simulink model "peacockElettricaSimulink"  (R2026a)
settings: Solver=FixedStepAuto  StopTime=40  FixedStep=0.001  EnableMultiTasking=on
InitFcn:
  | run('setupParams.m');
  | %run("tracks\track2.m");
StopFcn:
  | plot(out.X, out.Y);
  | axis equal;
  | grid on;
model workspace: external: MATLAB File (data not in the file)
values from neighbouring files (symbols this model uses):
  aero_bal_r = 0.5    [setupParams.m]    (also in setupParamsSingle.m)
  Af = 1.1    [setupParams.m]    (also in setupParamsSingle.m)
  auto_speed = 0    [setupParams.m]
  ay_limit = 15.0    (= 15)    [setupParams.m]    (also in setupParamsSingle.m)
  brake_bias_f = 0.40    (= 0.4)    [setupParams.m]    (also in setupParamsSingle.m = 0.6)
  brake_bias_r = 1 - brake_bias_f    (= 0.6)    [setupParams.m]    (also in setupParamsSingle.m = 0.4)
  camber_front = -1.5    [setupParams.m]    (also in setupParamsSingle.m)
  camber_rear = -1    [setupParams.m]    (also in setupParamsSingle.m)
  Cl = 1.0    (= 1)    [setupParams.m]    (also in setupParamsSingle.m)
  deathzone_APP = 5    [setupParams.m]    (also in setupParamsSingle.m)
  e_yaw_deadzone = 0.03    [setupParams.m]
  falling_slew_rate_torque = -500    [setupParams.m]    (also in setupParamsSingle.m)
  g = 9.81    [setupParams.m]    (also in setupParamsSingle.m)
  gnd_displ = 0.0    (= 0)    [setupParams.m]    (also in setupParamsSingle.m)
  h_o = 0.35    [setupParams.m]    (also in setupParamsSingle.m)
  I_charge_max = 21    [setupParams.m]
  I_discharge_max = 90    [setupParams.m]
  K_roll_rear = 0.6    [setupParams.m]    (also in setupParamsSingle.m = 0.5)
  Kus = 0.03    [setupParams.m]    (also in setupParamsSingle.m = 0)
  l_f = 0.775    [setupParams.m]    (also in setupParamsSingle.m)
  l_r = 0.775    [setupParams.m]    (also in setupParamsSingle.m)
  launch_ramp_rate = 1000.0    (= 1000)    [setupParams.m]    (also in setupParamsSingle.m)
  launch_V_thresh = 5.0    (= 5)    [setupParams.m]    (also in setupParamsSingle.m)
  mass = 320    [setupParams.m]    (also in setupParamsSingle.m = 300)
  mu = 1.5    [setupParams.m]    (also in setupParamsSingle.m)
  nominal_ramp_rate = 1000.0    (= 1000)    [setupParams.m]    (also in setupParamsSingle.m)
  overslip_factor = 1.01    [setupParams.m]    (also in setupParamsSingle.m = 1.13)
  pa_front_wheel = 82700    [setupParams.m]    (also in setupParamsSingle.m)
  pa_rear_wheel = 82700    [setupParams.m]    (also in setupParamsSingle.m)
  pedal_bp = (0:10:100)'    [setupParams.m]    (also in setupParamsSingle.m)
  pedal_map = (pedal_bp / 100) .^ pedal_alpha    [setupParams.m]    (also in setupParamsSingle.m = (pedal_bp / 100) .^ pedal_alpha.Value)
  R_wheel = 0.2032    [setupParams.m]    (also in setupParamsSingle.m)
  regen_I_cont_A = 14.0    (= 14)    [setupParams.m]    (also in setupParamsSingle.m)
  regen_I_peak_A = 21.0    (= 21)    [setupParams.m]    (also in setupParamsSingle.m)
  regen_I_peak_dur_s = 4.0    (= 4)    [setupParams.m]    (also in setupParamsSingle.m)
  regen_P_batt_max_W = 35000    [setupParams.m]    (also in setupParamsSingle.m)
  regen_pedal_thr = 5.0    (= 5)    [setupParams.m]    (also in setupParamsSingle.m = 10)
  regen_speed_crit_rpm = 1000    [setupParams.m]    (also in setupParamsSingle.m = 500)
  regen_speed_min_rpm = 4000    [setupParams.m]    (also in setupParamsSingle.m = 3000)
  regen_T_max = 9    [setupParams.m]    (also in setupParamsSingle.m = Simulink.Parameter(T_rated.Value/2))
  rho = 1.225    [setupParams.m]    (also in setupParamsSingle.m)
  rid_eff = 0.80    (= 0.8)    [setupParams.m]    (also in setupParamsSingle.m)
  rid_ratio = 15    [setupParams.m]    (also in setupParamsSingle.m)
  rising_slew_rate_torque = 100    [setupParams.m]    (also in setupParamsSingle.m)
  rpm_safe_threshold = 100    [setupParams.m]
  scale_factor_front = ones(27, 1)    [setupParams.m]    (also in setupParamsSingle.m)
  scale_factor_rear = ones(27, 1)    [setupParams.m]    (also in setupParamsSingle.m)
  slip_bc_coeff = 10    [setupParams.m]    (also in setupParamsSingle.m = Simulink.Parameter(1.5))
  slip_filt_N = 80    [setupParams.m]    (also in setupParamsSingle.m = 15)
  slip_Kd = 0.8    [setupParams.m]    (also in setupParamsSingle.m = Simulink.Parameter(5.0))
  slip_Ki = 13.0    (= 13)    [setupParams.m]    (also in setupParamsSingle.m = Simulink.Parameter(110.0))
  slip_Kp = 50.0    (= 50)    [setupParams.m]    (also in setupParamsSingle.m = Simulink.Parameter(180.0))
  slip_low_sat = 0.0    (= 0)    [setupParams.m]    (also in setupParamsSingle.m)
  slip_ref = 0.15    [setupParams.m]    (also in setupParamsSingle.m = Simulink.Parameter(0.15))
  slip_up_sat = 25    [setupParams.m]    (also in setupParamsSingle.m = 21)
  slip_V_min = 3    [setupParams.m]    (also in setupParamsSingle.m = 1)
  steer_ratio = 4.2    [pure_pursuit.m]    (also in setupParams.m; setupParamsSingle.m)
  steering_deadband = 1    [setupParams.m]
  T_headroom_k = 13.0    (= 13)    [setupParams.m]    (also in setupParamsSingle.m = Simulink.Parameter(5.0))
  T_headroom_max = 9    [setupParams.m]    (also in setupParamsSingle.m = Simulink.Parameter(5.0))
  T_peak = 20    [setupParams.m]    (also in setupParamsSingle.m = 21)
  T_rated = 9.8    [setupParams.m]    (also in setupParamsSingle.m = Simulink.Parameter(9.8))
  track_width = (track_width_r + track_width_f)/2    (= 1.2)    [setupParams.m]    (also in setupParamsSingle.m = sqrt(track_width_r^2 + track_width_f^2))
  track_width_f = 1.2    [setupParams.m]    (also in setupParamsSingle.m)
  track_width_r = 1.2    [setupParams.m]    (also in setupParamsSingle.m)
  Ts = 0.01    [setupParams.m]    (also in setupParamsSingle.m)
  tvc_bc = 17    [setupParams.m]
  tvc_D_thresh = 0.060    (= 0.06)    [setupParams.m]    (also in setupParamsSingle.m)
  tvc_D_thresh_off = 0.03    [setupParams.m]    (also in setupParamsSingle.m)
  tvc_Kd = 100    [setupParams.m]    (also in setupParamsSingle.m = Simulink.Parameter(5))
  tvc_Ki = 150    [setupParams.m]    (also in setupParamsSingle.m = Simulink.Parameter(10))
  tvc_Kp = 650    [setupParams.m]    (also in setupParamsSingle.m = Simulink.Parameter(70))
  tvc_N_filter = 25    [setupParams.m]    (also in setupParamsSingle.m = Simulink.Parameter(20))
  tvc_sat_dMz = 700    [setupParams.m]    (also in setupParamsSingle.m = Simulink.Parameter(10.0))
  tvc_throttle_on = 3.0    (= 3)    [setupParams.m]    (also in setupParamsSingle.m = Simulink.Parameter(3.0))
  tvc_tr = 5    [setupParams.m]    (also in setupParamsSingle.m = Simulink.Parameter(1.0))
  tvc_V_off = 2.0    (= 2)    [setupParams.m]    (also in setupParamsSingle.m = Simulink.Parameter(2.0))
  tvc_V_on = 4.0    (= 4)    [setupParams.m]    (also in setupParamsSingle.m = Simulink.Parameter(4.0))
  tvc_yaw_thresh = 0.08    [setupParams.m]    (also in setupParamsSingle.m)
  tvc_yaw_thresh_off = 0.04    [setupParams.m]    (also in setupParamsSingle.m)
  V_dc = 540    [setupParams.m]    (also in setupParamsSingle.m)
  w_engine = 0.005    [setupParams.m]    (also in setupParamsSingle.m)
  wheelbase = l_f + l_r    (= 1.55)    [setupParams.m]    (also in setupParamsSingle.m)
undefined symbols (not defined in the file or in its folder): V_ref, X_ref, Y_ref
libraries: simulink x74, slpidlib x8, vehdynlibtire x8, dspsigops x4, vehdynlibsteering x2, autolibshared x2, sim3dautolib x2, sim3dlib x1, robotalgslib x1
(part 6 of 6)

== matlab function peacockElettricaSimulink/DriveController_/TVC/TorqueAllocator ==
  data: T_req input; T_RL_cmd output; dT input; n_motorRL input; n_motorRR input; T_RR_cmd output; D input; V_dc parameter; T_peak parameter; T_headroom_max parameter; T_headroom_k parameter; T_grip_max_RL input; T_grip_max_RR input; rpm_safe_threshold parameter; I_discharge_max parameter
function [T_RL_cmd, T_RR_cmd] = fcn(T_req, dT, n_motorRL, n_motorRR, D, ...
    V_dc, T_peak, T_headroom_max, T_headroom_k, T_grip_max_RL, T_grip_max_RR, rpm_safe_threshold, I_discharge_max)
    T_min = 0;
    
    % --- CALCOLO POTENZA MASSIMA (Inverter) ---
    P_max_inverter = V_dc * 58.33; 
    
    % --- CALCOLO LIMITI ELETTRICI (FIELD WEAKENING) ---
    w_RL = max(abs(n_motorRL) * (pi/30), 1.0); 
    w_RR = max(abs(n_motorRR) * (pi/30), 1.0);
    
    T_fw_L = P_max_inverter / w_RL;
    T_fw_R = P_max_inverter / w_RR;
    
    T_elec_max_RL = min(T_peak, T_fw_L);
    T_elec_max_RR = min(T_peak, T_fw_R);
    
    % --- LIMITI FISICI GLOBALI ---
    T_max_L = min(T_elec_max_RL, T_grip_max_RL);
    T_max_R = min(T_elec_max_RR, T_grip_max_RR);
    
    % ---  PROTEZIONE ASIMMETRIA E HEADROOM TVC ---
    T_lim_base = min(T_max_L, T_max_R);
    T_headroom = min(T_headroom_max, T_headroom_k * abs(D));
    
    T_lim_base_neg = -min(T_grip_max_RL, T_grip_max_RR); 
    
    if T_req >= 0
        T_req_eff = max(0, min(T_req, T_lim_base - T_headroom));
    else
        T_req_eff = max(T_lim_base_neg + T_headroom, min(0, T_req));
    end
    
    % ---  TEORICO TVC ---
    T_L = T_req_eff - dT;
    T_R = T_req_eff + dT;
    
    if (abs(n_motorRL) < rpm_safe_threshold) && (T_L < 0)
        T_L = 0;
    end
    if (abs(n_motorRR) < rpm_safe_threshold) && (T_R < 0)
        T_R = 0;
    end
    
    % --- LIMITAZIONE PROPORZIONALE POTENZA DC (DC Current Limit) ---
    P_req_L = max(0, T_L * w_RL);
    P_req_R = max(0, T_R * w_RR);
    P_tot_req = P_req_L + P_req_R;
    
    P_limit_dc = V_dc * I_discharge_max;
    
    if P_tot_req > P_limit_dc
        scale_factor = P_limit_dc / P_tot_req;
        T_L = T_L * scale_factor;
        T_R = T_R * scale_factor;
    end
    
    % --- SATURAZIONE FINALE ---
    T_RL_cmd = max(-T_grip_max_RL, min(T_max_L, T_L));
    T_RR_cmd = max(-T_grip_max_RR, min(T_max_R, T_R));
end

== matlab function peacockElettricaSimulink/G_motor_RR/MATLAB Function ==
  data: T_thermal input; T_req input; derating_out output; derating_prev input; derating_on_thresh parameter
% function derating_out = fcn(T_thermal, derating_prev,T_peak, derating_on_thresh, derating_off_thresh)
%     if derating_prev == 0
%         % Se il limite termico cala troppo, attivo il flag
%         derating_out = double(T_thermal < derating_on_thresh);
%     else
%         % Resto in derating finché il limite non ha recuperato abbastanza
%         derating_out = double(T_thermal < derating_off_thresh);
%     end
% end

function derating_out = fcn(T_thermal, T_req, derating_prev,derating_on_thresh)

if derating_prev == 0
    % Se NON sono in derating, controllo se devo entrarci
    if T_thermal < derating_on_thresh
        derating_out = 1;
    else
        derating_out = 0;
    end
else
    if T_req <= 1 % Uso un piccolo margine invece di 0 spaccato per robustezza numerica
        derating_out = 0; % Esco dal derating
    else
        derating_out = 1; % Mantengo il derating
    end
end
end

== matlab function peacockElettricaSimulink/DriveController_/Yaw_th/tand safe ==
  data: tand input; tand_safe output; angle_limit_d parameter
function tand_safe = fcn(tand,angle_limit_d)
    soglia = tan(angle_limit_d*pi/180);  % 2° rad
    
    if abs(tand) < soglia
        tand_safe = 0;  % 
    else
        tand_safe = tand;  
    end
end

== matlab function peacockElettricaSimulink/DriveController_/Yaw_th/yaw_saturation ==
  data: yaw_th input; yaw_sat output; V input; mu parameter; g parameter
function yaw_sat = fcn(yaw_th, V,mu, g)
    V_calc = max(V, 0.5);
    
    yaw_max_abs = (mu * g) / V_calc;
    yaw_sat = sign(yaw_th) * min(abs(yaw_th), yaw_max_abs);
end

== matlab function peacockElettricaSimulink/DriveController_/SRC/MATLAB Function ==
  data: enable input; T_cut_RL output; Delta_T_raw input
function T_cut_RL = fcn(enable, Delta_T_raw)
    T_cut_RL = enable * Delta_T_raw;
end

== matlab function peacockElettricaSimulink/DriveController_/SRC/MATLAB Function1 ==
  data: enable input; T_cut_RR output; Delta_T_raw input
function T_cut_RR = fcn(enable, Delta_T_raw)
    T_cut_RR = enable * Delta_T_raw;
end

== matlab function peacockElettricaSimulink/PeacockElettrica_/MATLAB Function1 ==
  data: Vx input; Vx_hub output; Vy input; yaw input; delta_L input; delta_R input; Vy_hub output; track_width_f parameter; track_width_r parameter; l_f parameter; l_r parameter
function [Vx_hub, Vy_hub] = wheel_kinematics(Vx, Vy, yaw, delta_L, delta_R, track_width_f, track_width_r, l_f, l_r)
% Trasforma le velocità del baricentro (CG) nelle velocità locali dei mozzi ruota.
%
% INPUTS:
% Vx, Vy  : Velocità longitudinali e laterali del veicolo (CG) [m/s]
% yaw       : Velocità di imbardata (Yaw rate) [rad/s]
% delta_L : Angolo di sterzo ruota anteriore sinistra [rad]
% delta_R : Angolo di sterzo ruota anteriore destra [rad]
% l_f, l_r: Distanza baricentro - asse anteriore/posteriore [m]
% track_width_f, track_width_r: Carreggiata (Track width) anteriore/posteriore [m]
%
% OUTPUTS:
% Vx_hub  : Vettore [FL, FR, RL, RR] delle velocità longitudinali dei mozzi [m/s]
% Vy_hub  : Vettore [FL, FR, RL, RR] delle velocità laterali dei mozzi [m/s]

    %% 1. Velocità nel sistema di riferimento del telaio (non ruotate)
    % Anteriore Sinistra (Front Left)
    V_xf_FL = Vx - (yaw * track_width_f / 2);
    V_yf_FL = Vy + (yaw * l_f);
    
    % Anteriore Destra (Front Right)
    V_xf_FR = Vx + (yaw * track_width_f / 2);
    V_yf_FR = Vy + (yaw * l_f);
    
    % Posteriore Sinistra (Rear Left)
    V_xr_RL = Vx - (yaw * track_width_r / 2);
    V_yr_RL = Vy - (yaw * l_r);
    
    % Posteriore Destra (Rear Right)
    V_xr_RR = Vx + (yaw * track_width_r / 2);
    V_yr_RR = Vy - (yaw * l_r);

    %% 2. Rotazione nel sistema di riferimento della gomma (tramite angolo di sterzo)
    % Le ruote anteriori sono sterzanti
    Vx_FL =  V_xf_FL * cos(delta_L) + V_yf_FL * sin(delta_L);
    Vy_FL = -V_xf_FL * sin(delta_L) + V_yf_FL * cos(delta_L);
    
    Vx_FR =  V_xf_FR * cos(delta_R) + V_yf_FR * sin(delta_R);
    Vy_FR = -V_xf_FR * sin(delta_R) + V_yf_FR * cos(delta_R);
    
    % Le ruote posteriori solitamente non sterzano (delta = 0, quindi cos(0)=1, sin(0)=0)
    Vx_RL = V_xr_RL;
    Vy_RL = V_yr_RL;
    
    Vx_RR = V_xr_RR;
    Vy_RR = V_yr_RR;

    Vx_hub = [Vx_FL; Vx_FR; Vx_RL; Vx_RR];
    Vy_hub = [Vy_FL; Vy_FR; Vy_RL; Vy_RR];
end

== matlab function peacockElettricaSimulink/DriveController_/MATLAB Function ==
  settings: updateMethod=DISCRETE
  data: throttle_pct input; T_regen output; n_motorRL input; n_motorRR input; V input; regen_active output; Ts parameter; regen_T_max parameter; regen_pedal_thr parameter; regen_speed_min_rpm parameter; regen_speed_crit_rpm parameter; regen_I_peak_A parameter; regen_I_cont_A parameter; regen_I_peak_dur_s parameter; regen_P_batt_max_W parameter; V_dc parameter; ay input; ay_limit parameter; I_charge_max parameter
function [T_regen, regen_active] = regen_fcn( ...
        throttle_pct, n_motorRL, n_motorRR, V, Ts, ...
        regen_T_max, regen_pedal_thr, regen_speed_min_rpm, regen_speed_crit_rpm, ...
        regen_I_peak_A, regen_I_cont_A, regen_I_peak_dur_s, ...
        regen_P_batt_max_W, V_dc, ay, ay_limit, I_charge_max)

    persistent t_elapsed_s;
    if isempty(t_elapsed_s)
        t_elapsed_s = 0.0;
    end
    speed_avg_rpm = (abs(n_motorRL) + abs(n_motorRR)) * 0.5;
    
    % ---- condizione di abilitazione regen 
    should_regen = (throttle_pct <= regen_pedal_thr) && ...
                   (speed_avg_rpm > regen_speed_crit_rpm) && ...
                   (V > 0.5);
    if ~should_regen
        t_elapsed_s = 0.0;
        T_regen = 0;
        regen_active = 0.0;
        return;
    end
    
    t_elapsed_s = t_elapsed_s + Ts;
    
    % ---- Stage 1: coppia pedal-dipendente [Nm, negativa] ----------------
    pedal_norm = throttle_pct / regen_pedal_thr;
    T_s1 = -regen_T_max * (1.0 - pedal_norm);
    
    % ---- Stage 2: fade-out velocità -------------------------------------
    if speed_avg_rpm >= regen_speed_min_rpm
        k_vel = 1.0;
    else
        k_vel = speed_avg_rpm / regen_speed_min_rpm;
    end
    T_s2 = T_s1 * k_vel;
    
    % ---- Stage 3: limite potenza batteria (per motore = totale/2) -------
    omega_rad_s = (2.0 * pi * speed_avg_rpm) / 60.0;
    omega_safe  = max(omega_rad_s, 1.0);          
    T_P_lim     = (regen_P_batt_max_W * 0.5) / omega_safe;
    T_s3        = max(T_s2, -T_P_lim);            
    
    % --- NUOVO: INCROCIO LIMITI DI CORRENTE BMS ---
    if t_elapsed_s < regen_I_peak_dur_s
        I_lim_teorico = regen_I_peak_A;    
    else
        I_lim_teorico = regen_I_cont_A;   
    end
    
    % Sceglie il limite più severo tra la logica timer e il CAN del BMS
    I_lim_effettivo = min(I_lim_teorico, I_charge_max);
    I_lim_per_mot = I_lim_effettivo * 0.5;
    
    T_I_lim = (I_lim_per_mot * V_dc) / omega_safe;
    T_final = max(T_s3, -T_I_lim);
    
    % ---- Stage 4: limite regen x curva ----------------------------------
    k_derating_ay = max(0.0, 1.0 - (abs(ay) / ay_limit));
    T_final = T_final * k_derating_ay;
    
    % ---- output simmetrico sui due motori -------------------------------
    T_regen  = T_final;
    regen_active = 1; 
end

== matlab function peacockElettricaSimulink/DriveController_/MATLAB Function1 ==
  data: T_max_RL output; v_x input; a_x input; a_y input; T_max_RR output; mass parameter; g parameter; wheelbase parameter; l_f parameter; track_width_r parameter; mu parameter; h_o parameter; R_wheel parameter; Af parameter; Cl parameter; aero_bal_r parameter; K_roll_rear parameter; rho parameter; rid_ratio parameter; rid_eff parameter; overslip_factor parameter
function [T_max_RL, T_max_RR] = GripEstimator(v_x, a_x, a_y, mass, g, wheelbase, l_f, track_width_r,mu,h_o, R_wheel,Af, Cl, aero_bal_r, K_roll_rear, rho, rid_ratio,rid_eff, overslip_factor)
    % ---------------------------------------------------------
    % 1. CARICO BASE (Statico + Aerodinamico)
    % ---------------------------------------------------------
    Fz_stat_rear = mass * g * (l_f / wheelbase);
    
    Fz_aero_rear = 0.5 * rho * Af * Cl * (v_x^2) * aero_bal_r;
    
    Fz_base_wheel = (Fz_stat_rear + Fz_aero_rear) / 2;

   
    % 2. TRASFERIMENTI DI CARICO
    % Longitudinale: se a_x > 0 (accelerazione), il peso si sposta dietro (+)
    delta_Fz_long = 0.5 * (mass * a_x * h_o / wheelbase);
    
    % Laterale: dipende dall'accelerazione laterale a_y.
    % Convenzione: a_y < 0 per curva a destra-> peso si sposta a sinistra.
    delta_Fz_lat = (mass * a_y * h_o / track_width_r) * K_roll_rear;

    % 3. FORZE NORMALI FINALI SULLE RUOTE (Fz)
    Fz_RL = Fz_base_wheel + delta_Fz_long + delta_Fz_lat;
    Fz_RR = Fz_base_wheel + delta_Fz_long - delta_Fz_lat;

    % Prevenzione valori negativi (se la ruota interna si alza da terra, Fz = 0)
    if Fz_RL < 0
        Fz_RL = 0;
    end
    if Fz_RR < 0
        Fz_RR = 0;
    end
    

    
    % 4. CALCOLO COPPIA MASSIMA AI MOTORI
    % T = (F * R) / (tau * eff)

    % Parametri Pacejka (dal file .tir)
    Fz0 = 1112.0;
    PDX1 = 1.00347;
    PDX2 = -0.99198;

    % Calcolo mu dinamico per lato sinistro
    dfz_RL = (Fz_RL - Fz0) / Fz0;
    mu_RL = PDX1 + (PDX2 * dfz_RL);
    
    % Saturazione di sicurezza (evita mu negativi o assurdi)
    if mu_RL < 0.5; mu_RL = 0.5; end

    % Calcolo mu dinamico per lato destro
    dfz_RR = (Fz_RR - Fz0) / Fz0;
    mu_RR = PDX1 + (PDX2 * dfz_RR);
    if mu_RR < 0.5; mu_RR = 0.5; end
    
   

    % % Calcolo coppia massima ai motori usando il mu corretto
    % T_max_RL = (Fz_RL * mu_RL * R_wheel) / (rid_ratio * rid_eff);
    % T_max_RR = (Fz_RR * mu_RR * R_wheel) / (rid_ratio * rid_eff);

    % Calcolo coppia massima ai motori
     %T_max_RL = ((Fz_RL * mu_RL * R_wheel) / (rid_ratio * rid_eff)) * overslip_factor;
     %T_max_RR = ((Fz_RR * mu_RR * R_wheel) / (rid_ratio * rid_eff)) * overslip_factor;

    T_max_RL = (Fz_RL * mu * R_wheel) / (rid_ratio * rid_eff)* overslip_factor;
    T_max_RR = (Fz_RR * mu * R_wheel) / (rid_ratio * rid_eff)* overslip_factor;
end

== matlab function peacockElettricaSimulink/G_motor_RR/MATLAB Function1 ==
  data: rpm_motor input; T_limit output; V_dc input
function T_limit = fcn(rpm_motor, V_dc)
    %potenza massima erogabile: 35kW(max) / 600V = 58.33
    P_max = V_dc * 58.33; 

    w_rad = max(abs(rpm_motor) * (pi/30), 1.0); 

    T_limit = P_max / w_rad;
end

== matlab function peacockElettricaSimulink/G_motor_RL/Field weakening ==
  data: rpm_motor input; T_limit output; V_dc input
function T_limit = fcn(rpm_motor, V_dc)
    P_max = V_dc * 58.33; 

    w_rad = max(abs(rpm_motor) * (pi/30), 1.0); 

    T_limit = P_max / w_rad;
end

== matlab function peacockElettricaSimulink/PeacockElettrica_/MATLAB Function ==
  data: Fx_FL input; FwF output; Fy_FL input; Fx_FR input; Fy_FR input; Fx_RL input; Fy_RL input; Fx_RR input; Fy_RR input; delta_L input; FwR output; delta_R input
function [FwF, FwR] = rotazione_forze(Fx_FL, Fy_FL, Fx_FR, Fy_FR, Fx_RL, Fy_RL, Fx_RR, Fy_RR, delta_L, delta_R)
    
    % 1. Ruota le forze della ruota Anteriore Sinistra (FL) usando l'angolo sinistro (delta_L)
    Fx_veh_FL = Fx_FL * cos(delta_L) - Fy_FL * sin(delta_L);
    Fy_veh_FL = Fx_FL * sin(delta_L) + Fy_FL * cos(delta_L);

    % 2. Ruota le forze della ruota Anteriore Destra (FR) usando l'angolo destro (delta_R)
    Fx_veh_FR = Fx_FR * cos(delta_R) - Fy_FR * sin(delta_R);
    Fy_veh_FR = Fx_FR * sin(delta_R) + Fy_FR * cos(delta_R);

    % 3. Crea la matrice 2x2 per la porta FwF (Asse Anteriore)
    FwF = [Fx_veh_FL, Fy_veh_FL;
           Fx_veh_FR, Fy_veh_FR];

    % 4. Crea la matrice 2x2 per la porta FwR (Asse Posteriore)
    % (Le posteriori non sterzano, quindi i valori rimangono quelli originali della gomma)
    FwR = [Fx_RL, Fy_RL;
           Fx_RR, Fy_RR];
end

== matlab function peacockElettricaSimulink/MATLAB Function ==
  data: curv input; v_curv output; a_lat_max parameter
function v_curv = fcn(curv,a_lat_max)

v_curv_raw = sqrt(a_lat_max / (abs(curv)+0.001));

v_curv = min(v_curv_raw, 100);

== matlab function peacockElettricaSimulink/Target Velocity Profiler ==
  data: x input; V_target output; y input; lookahead_pts input; X_ref parameter; Y_ref parameter; V_ref parameter
function V_target = fcn(x, y, lookahead_pts, X_ref, Y_ref, V_ref)
    % V_TARGET_PROFILER Trova la velocità target in base alla posizione
    % X_ref, Y_ref, V_ref_array devono essere passati come Parametri (o segnali) di dimensione [1x1500]
    
    % 1. Calcola la distanza quadrata tra l'auto e tutti i punti della traiettoria
    dist_sq = (X_ref - x).^2 + (Y_ref - y).^2;
    
    % 2. Trova l'indice del punto più vicino sulla pista
    [~, current_idx] = min(dist_sq);
    
    % 3. Look-ahead della velocità (FONDAMENTALE PER LA FRENATA)
    % Se chiedi all'auto di rallentare quando è GIA' nel punto di corda, andrà dritta.
    % Dobbiamo dirle di guardare la velocità dei punti successivi per iniziare a frenare prima.
    target_idx = current_idx + lookahead_pts;
    
    % Gestione della chiusura del tracciato (loop)
    num_points = length(X_ref);
    if target_idx > num_points
        target_idx = target_idx - num_points; 
    end
    
    % 4. Estrai la velocità di riferimento
    V_target = V_ref(target_idx);
end

== matlab function peacockElettricaSimulink/PeacockElettrica/Car Body/MATLAB Function ==
  data: delta_L input; delta_R input; Fx_FL input; FwF output; Fy_FL input; Fx_FR input; Fy_FR input; Fx_RL input; Fy_RL input; Fx_RR input; Fy_RR input; FwR output
function [FwF, FwR] = rotationary_forces(delta_L, delta_R, Fx_FL, Fy_FL, Fx_FR, Fy_FR, Fx_RL, Fy_RL, Fx_RR, Fy_RR)
    
    % 1. Ruota le forze della ruota Anteriore Sinistra (FL) usando l'angolo sinistro (delta_L)
    Fx_veh_FL = Fx_FL * cos(delta_L) - Fy_FL * sin(delta_L);
    Fy_veh_FL = Fx_FL * sin(delta_L) + Fy_FL * cos(delta_L);

    % 2. Ruota le forze della ruota Anteriore Destra (FR) usando l'angolo destro (delta_R)
    Fx_veh_FR = Fx_FR * cos(delta_R) - Fy_FR * sin(delta_R);
    Fy_veh_FR = Fx_FR * sin(delta_R) + Fy_FR * cos(delta_R);


FwF = [Fx_veh_FL, -Fy_veh_FL;
       Fx_veh_FR, -Fy_veh_FR];

FwR = [Fx_RL, -Fy_RL;
       Fx_RR, -Fy_RR];
end

== matlab function peacockElettricaSimulink/DriveController_/TVC/MATLAB Function ==
  data: dMz input; dT output; R_wheel parameter; track_width parameter; rid_ratio parameter; rid_eff parameter
function dT = fcn(dMz, R_wheel, track_width, rid_ratio, rid_eff)
    dT = dMz * R_wheel / (track_width * rid_ratio * rid_eff);
end

== matlab function peacockElettricaSimulink/PeacockElettrica/Car Body/car2wheels ==
  data: delta_L input; delta_R input; Vx input; Vx_hub output; Vy input; yaw_rate input; Vy_hub output; track_width_f parameter; track_width_r parameter; l_f parameter; l_r parameter
function [Vx_hub, Vy_hub] = wheel_kinematics(delta_L, delta_R, Vx, Vy, yaw_rate, track_width_f, track_width_r, l_f, l_r)
% Trasforma le velocità del baricentro (CG) nelle velocità locali dei mozzi ruota.
%
% INPUTS:
% Vx, Vy  : Velocità longitudinali e laterali del veicolo (CG) [m/s]
% yaw_rate       : Velocità di imbardata (yaw_rate ) [rad/s]
% delta_L : Angolo di sterzo ruota anteriore sinistra [rad]
% delta_R : Angolo di sterzo ruota anteriore destra [rad]
% l_f, l_r: Distanza baricentro - asse anteriore/posteriore [m]
% track_width_f, track_width_r: Carreggiata (Track width) anteriore/posteriore [m]
%
% OUTPUTS:
% Vx_hub  : Vettore [FL, FR, RL, RR] delle velocità longitudinali dei mozzi [m/s]
% Vy_hub  : Vettore [FL, FR, RL, RR] delle velocità laterali dei mozzi [m/s]

    %% 1. Velocità nel sistema di riferimento del telaio (non ruotate)
    % Anteriore Sinistra (Front Left)
    V_xf_FL = Vx - (yaw_rate * track_width_f / 2);
    V_yf_FL = Vy + (yaw_rate * l_f);
    
    % Anteriore Destra (Front Right)
    V_xf_FR = Vx + (yaw_rate * track_width_f / 2);
    V_yf_FR = Vy + (yaw_rate * l_f);
    
    % Posteriore Sinistra (Rear Left)
    V_xr_RL = Vx - (yaw_rate * track_width_r / 2);
    V_yr_RL = Vy - (yaw_rate * l_r);
    
    % Posteriore Destra (Rear Right)
    V_xr_RR = Vx + (yaw_rate * track_width_r / 2);
    V_yr_RR = Vy - (yaw_rate * l_r);

    %% 2. Rotazione nel sistema di riferimento della gomma (tramite angolo di sterzo)
    % Le ruote anteriori sono sterzanti
    Vx_FL =  V_xf_FL * cos(delta_L) + V_yf_FL * sin(delta_L);
    Vy_FL = -V_xf_FL * sin(delta_L) + V_yf_FL * cos(delta_L);
    
    Vx_FR =  V_xf_FR * cos(delta_R) + V_yf_FR * sin(delta_R);
    Vy_FR = -V_xf_FR * sin(delta_R) + V_yf_FR * cos(delta_R);
    
    % Le ruote posteriori solitamente non sterzano (delta = 0, quindi cos(0)=1, sin(0)=0)
    Vx_RL = V_xr_RL;
    Vy_RL = V_yr_RL;
    
    Vx_RR = V_xr_RR;
    Vy_RR = V_yr_RR;

    Vx_hub = [Vx_FL; Vx_FR; Vx_RL; Vx_RR];
    Vy_hub = [Vy_FL; Vy_FR; Vy_RL; Vy_RR];
end

== matlab function peacockElettricaSimulink/PeacockElettrica/G_motor_RL/Derating ==
  data: T_thermal input; T_req input; derating_out output; derating_prev input; derating_on_thresh parameter
function derating_out = fcn(T_thermal, T_req, derating_prev,derating_on_thresh)

if derating_prev == 0
    % Se NON sono in derating, controllo se devo entrarci
    if T_thermal < derating_on_thresh
        derating_out = 1;
    else
        derating_out = 0;
    end
else
    if T_req <= 1 % Uso un piccolo margine invece di 0 spaccato per robustezza numerica
        derating_out = 0; % Esco dal derating
    else
        derating_out = 1; % Mantengo il derating
    end
end
end

== matlab function peacockElettricaSimulink/PeacockElettrica/G_motor_RL/Field weakening ==
  data: rpm_motor input; T_limit output; V_dc input
function T_limit = fcn(rpm_motor, V_dc)
    P_max = V_dc * 58.33; 

    w_rad = max(abs(rpm_motor) * (pi/30), 1.0); 

    T_limit = P_max / w_rad;
end

== matlab function peacockElettricaSimulink/PeacockElettrica/G_motor_RR/MATLAB Function ==
  data: T_thermal input; T_req input; derating_out output; derating_prev input; derating_on_thresh parameter
% function derating_out = fcn(T_thermal, derating_prev,T_peak, derating_on_thresh, derating_off_thresh)
%     if derating_prev == 0
%         % Se il limite termico cala troppo, attivo il flag
%         derating_out = double(T_thermal < derating_on_thresh);
%     else
%         % Resto in derating finché il limite non ha recuperato abbastanza
%         derating_out = double(T_thermal < derating_off_thresh);
%     end
% end

function derating_out = fcn(T_thermal, T_req, derating_prev,derating_on_thresh)

if derating_prev == 0
    % Se NON sono in derating, controllo se devo entrarci
    if T_thermal < derating_on_thresh
        derating_out = 1;
    else
        derating_out = 0;
    end
else
    if T_req <= 1 % Uso un piccolo margine invece di 0 spaccato per robustezza numerica
        derating_out = 0; % Esco dal derating
    else
        derating_out = 1; % Mantengo il derating
    end
end
end

== matlab function peacockElettricaSimulink/PeacockElettrica/G_motor_RR/MATLAB Function1 ==
  data: rpm_motor input; T_limit output; V_dc input
function T_limit = fcn(rpm_motor, V_dc)
    %potenza massima erogabile: 35kW(max) / 600V = 58.33
    P_max = V_dc * 58.33; 

    w_rad = max(abs(rpm_motor) * (pi/30), 1.0); 

    T_limit = P_max / w_rad;
end

== matlab function peacockElettricaSimulink/PeacockElettrica/Car Body/V ==
  data: Vx input; V output; Vy input
function V = fcn(Vx,Vy)

V = (Vx^2 + Vy^2)^0.5;

== matlab function peacockElettricaSimulink/DriveController/MATLAB Function ==
  settings: updateMethod=DISCRETE
  data: throttle_pct input; T_regen output; n_motorRL input; n_motorRR input; V input; regen_active output; Ts parameter; regen_T_max parameter; regen_pedal_thr parameter; regen_speed_min_rpm parameter; regen_speed_crit_rpm parameter; regen_I_peak_A parameter; regen_I_cont_A parameter; regen_I_peak_dur_s parameter; regen_P_batt_max_W parameter; V_dc parameter; ay input; ay_limit parameter; I_charge_max parameter
function [T_regen, regen_active] = regen_fcn( ...
        throttle_pct, n_motorRL, n_motorRR, V, Ts, ...
        regen_T_max, regen_pedal_thr, regen_speed_min_rpm, regen_speed_crit_rpm, ...
        regen_I_peak_A, regen_I_cont_A, regen_I_peak_dur_s, ...
        regen_P_batt_max_W, V_dc, ay, ay_limit, I_charge_max)

    persistent t_elapsed_s;
    if isempty(t_elapsed_s)
        t_elapsed_s = 0.0;
    end
    speed_avg_rpm = (abs(n_motorRL) + abs(n_motorRR)) * 0.5;
    
    % ---- condizione di abilitazione regen 
    should_regen = (throttle_pct <= regen_pedal_thr) && ...
                   (speed_avg_rpm > regen_speed_crit_rpm) && ...
                   (V > 0.5);
    if ~should_regen
        t_elapsed_s = 0.0;
        T_regen = 0;
        regen_active = 0.0;
        return;
    end
    
    t_elapsed_s = t_elapsed_s + Ts;
    
    % ---- Stage 1: coppia pedal-dipendente [Nm, negativa] ----------------
    pedal_norm = throttle_pct / regen_pedal_thr;
    T_s1 = -regen_T_max * (1.0 - pedal_norm);
    
    if n_motorRL < regen_speed_min_rpm || n_motorRR < regen_speed_min_rpm
        t_elapsed_s = 0.0;
        T_regen = 0;
        regen_active = 0.0;
        return;
    end
    % ---- Stage 2: fade-out velocità -------------------------------------
    if speed_avg_rpm >= regen_speed_min_rpm
        k_vel = 1.0;
    else
        k_vel = speed_avg_rpm / regen_speed_min_rpm;
    end
    T_s2 = T_s1 * k_vel;
    
    % ---- Stage 3: limite potenza batteria (per motore = totale/2) -------
    omega_rad_s = (2.0 * pi * speed_avg_rpm) / 60.0;
    omega_safe  = max(omega_rad_s, 1.0);          
    T_P_lim     = (regen_P_batt_max_W * 0.5) / omega_safe;
    T_s3        = max(T_s2, -T_P_lim);            
    
    % --- NUOVO: INCROCIO LIMITI DI CORRENTE BMS ---
    if t_elapsed_s < regen_I_peak_dur_s
        I_lim_teorico = regen_I_peak_A;    
    else
        I_lim_teorico = regen_I_cont_A;   
    end
    
    % Sceglie il limite più severo tra la logica timer e il CAN del BMS
    I_lim_effettivo = min(I_lim_teorico, I_charge_max);
    I_lim_per_mot = I_lim_effettivo * 0.5;
    
    T_I_lim = (I_lim_per_mot * V_dc) / omega_safe;
    T_final = max(T_s3, -T_I_lim);
    
    % ---- Stage 4: limite regen x curva ----------------------------------
    k_derating_ay = max(0.0, 1.0 - (abs(ay) / ay_limit));
    T_final = T_final * k_derating_ay;
    
    % ---- output simmetrico sui due motori -------------------------------
    T_regen  = T_final;
    regen_active = 1; 
end

== matlab function peacockElettricaSimulink/DriveController/MATLAB Function1 ==
  data: T_max_RL output; v_x input; a_x input; a_y input; T_max_RR output; mass parameter; g parameter; wheelbase parameter; l_f parameter; track_width_r parameter; mu parameter; h_o parameter; R_wheel parameter; Af parameter; Cl parameter; aero_bal_r parameter; K_roll_rear parameter; rho parameter; rid_ratio parameter; rid_eff parameter; overslip_factor parameter
function [T_max_RL, T_max_RR] = GripEstimator(v_x, a_x, a_y, mass, g, wheelbase, l_f, track_width_r,mu,h_o, R_wheel,Af, Cl, aero_bal_r, K_roll_rear, rho, rid_ratio,rid_eff, overslip_factor)
    % ---------------------------------------------------------
    % 1. CARICO BASE (Statico + Aerodinamico)
    % ---------------------------------------------------------
    Fz_stat_rear = mass * g * (l_f / wheelbase);
    
    Fz_aero_rear = 0.5 * rho * Af * Cl * (v_x^2) * aero_bal_r;
    
    Fz_base_wheel = (Fz_stat_rear + Fz_aero_rear) / 2;

   
    % 2. TRASFERIMENTI DI CARICO
    % Longitudinale: se a_x > 0 (accelerazione), il peso si sposta dietro (+)
    delta_Fz_long = 0.5 * (mass * a_x * h_o / wheelbase);
    
    % Laterale: dipende dall'accelerazione laterale a_y.
    % Convenzione: a_y < 0 per curva a destra-> peso si sposta a sinistra.
    delta_Fz_lat = (mass * a_y * h_o / track_width_r) * K_roll_rear;

    % 3. FORZE NORMALI FINALI SULLE RUOTE (Fz)
    Fz_RL = Fz_base_wheel + delta_Fz_long + delta_Fz_lat;
    Fz_RR = Fz_base_wheel + delta_Fz_long - delta_Fz_lat;

    % Prevenzione valori negativi (se la ruota interna si alza da terra, Fz = 0)
    if Fz_RL < 0
        Fz_RL = 0;
    end
    if Fz_RR < 0
        Fz_RR = 0;
    end
    

    
    % 4. CALCOLO COPPIA MASSIMA AI MOTORI
    % T = (F * R) / (tau * eff)

    % Parametri Pacejka (dal file .tir)
    Fz0 = 1112.0;
    PDX1 = 1.00347;
    PDX2 = -0.99198;

    % Calcolo mu dinamico per lato sinistro
    dfz_RL = (Fz_RL - Fz0) / Fz0;
    mu_RL = PDX1 + (PDX2 * dfz_RL);
    
    % Saturazione di sicurezza (evita mu negativi o assurdi)
    if mu_RL < 0.5; mu_RL = 0.5; end

    % Calcolo mu dinamico per lato destro
    dfz_RR = (Fz_RR - Fz0) / Fz0;
    mu_RR = PDX1 + (PDX2 * dfz_RR);
    if mu_RR < 0.5; mu_RR = 0.5; end
    
   

    % % Calcolo coppia massima ai motori usando il mu corretto
    % T_max_RL = (Fz_RL * mu_RL * R_wheel) / (rid_ratio * rid_eff);
    % T_max_RR = (Fz_RR * mu_RR * R_wheel) / (rid_ratio * rid_eff);

    % Calcolo coppia massima ai motori
     %T_max_RL = ((Fz_RL * mu_RL * R_wheel) / (rid_ratio * rid_eff)) * overslip_factor;
     %T_max_RR = ((Fz_RR * mu_RR * R_wheel) / (rid_ratio * rid_eff)) * overslip_factor;

    T_max_RL = (Fz_RL * mu * R_wheel) / (rid_ratio * rid_eff)* overslip_factor;
    T_max_RR = (Fz_RR * mu * R_wheel) / (rid_ratio * rid_eff)* overslip_factor;
end

== matlab function peacockElettricaSimulink/DriveController_/Yaw_th/Bicycle Model Dynamic ==
  data: V input; yaw_th output; tan_delta input; wheelbase parameter; Kus parameter
function yaw_th = fcn(V,tan_delta,wheelbase,Kus)
% L = 1.55; %passo veicolo [m]
% yaw_th = (V / L) * tand;
%
  
yaw_th = (V / wheelbase) * tan_delta / (1 + Kus * V^2);



end

== stateflow chart peacockElettricaSimulink/DriveController/Mode Manager ==
  state IDLE_
    entry:
    TVC_Target_Weight = 0;
  note: %[brake > 0 || (Throttle < tvc_throttle_on && V <= tvc_V_off)]
  state TVC_
    entry: TVC_Target_Weight = 1;
  (default) -> IDLE_
  TVC_ -> IDLE_ : [V <= tvc_V_off]
  IDLE_ -> TVC_ : [V > tvc_V_on]
  data: TVC_Target_Weight output; V input; D input; Throttle input; YawError input; brake input; tvc_D_thresh parameter; tvc_yaw_thresh parameter; tvc_yaw_thresh_off parameter; tvc_throttle_on parameter; tvc_V_on parameter; tvc_V_off parameter; tvc_D_thresh_off parameter

== matlab function peacockElettricaSimulink/DriveController/SRC/MATLAB Function ==
  data: enable input; T_cut_RL output; Delta_T_raw input
function T_cut_RL = fcn(enable, Delta_T_raw)
    T_cut_RL = enable * Delta_T_raw;
end

== matlab function peacockElettricaSimulink/DriveController/SRC/MATLAB Function1 ==
  data: enable input; T_cut_RR output; Delta_T_raw input
function T_cut_RR = fcn(enable, Delta_T_raw)
    T_cut_RR = enable * Delta_T_raw;
end

== matlab function peacockElettricaSimulink/DriveController/TVC/MATLAB Function ==
  data: dMz input; dT output; R_wheel parameter; track_width parameter; rid_ratio parameter; rid_eff parameter
function dT = fcn(dMz, R_wheel, track_width, rid_ratio, rid_eff)
    dT = dMz * R_wheel / (track_width * rid_ratio * rid_eff);
end

== matlab function peacockElettricaSimulink/DriveController/TVC/MATLAB Function1 ==
  data: dT_act input; dMz_act output; track_width parameter; R_wheel parameter; rid_ratio parameter; rid_eff parameter
function dMz_act = fcn(dT_act, track_width, R_wheel, rid_ratio, rid_eff)
    %Yaw moment (z) that the engines are currently delivering
    dMz_act = dT_act * track_width * rid_ratio * rid_eff / (2 * R_wheel);
end

== matlab function peacockElettricaSimulink/DriveController/TVC/TorqueAllocator ==
  data: T_req input; T_RL_cmd output; dT input; n_motorRL input; n_motorRR input; T_RR_cmd output; D input; V_dc parameter; T_peak parameter; T_headroom_max parameter; T_headroom_k parameter; T_grip_max_RL input; T_grip_max_RR input; rpm_safe_threshold parameter; I_discharge_max parameter
function [T_RL_cmd, T_RR_cmd] = fcn(T_req, dT, n_motorRL, n_motorRR, D, ...
    V_dc, T_peak, T_headroom_max, T_headroom_k, T_grip_max_RL, T_grip_max_RR, rpm_safe_threshold, I_discharge_max)
    T_min = 0;
    
    % --- CALCOLO POTENZA MASSIMA (Inverter) ---
    P_max_inverter = V_dc * 58.33; 
    
    % --- CALCOLO LIMITI ELETTRICI (FIELD WEAKENING) ---
    w_RL = max(abs(n_motorRL) * (pi/30), 1.0); 
    w_RR = max(abs(n_motorRR) * (pi/30), 1.0);
    
    T_fw_L = P_max_inverter / w_RL;
    T_fw_R = P_max_inverter / w_RR;
    
    T_elec_max_RL = min(T_peak, T_fw_L);
    T_elec_max_RR = min(T_peak, T_fw_R);
     
    % --- LIMITI FISICI GLOBALI ---
    T_max_L = min(T_elec_max_RL, T_grip_max_RL);
    T_max_R = min(T_elec_max_RR, T_grip_max_RR);
    
    % ---  PROTEZIONE ASIMMETRIA E HEADROOM TVC ---
    T_lim_base = min(T_max_L, T_max_R);
    T_headroom = min(T_headroom_max, T_headroom_k * abs(D));
    
    T_lim_base_neg = -min(T_grip_max_RL, T_grip_max_RR); 
    
    if T_req >= 0
        T_req_eff = max(0, min(T_req, T_lim_base - T_headroom));
    else
        T_req_eff = max(T_lim_base_neg + T_headroom, min(0, T_req));
    end
    
    % ---  TEORICO TVC ---
    T_L = T_req_eff - dT;
    T_R = T_req_eff + dT;
    
    if (abs(n_motorRL) < rpm_safe_threshold) && (T_L < 0)
        T_L = 0;
    end
    if (abs(n_motorRR) < rpm_safe_threshold) && (T_R < 0)
        T_R = 0;
    end
    
    % --- LIMITAZIONE PROPORZIONALE POTENZA DC (DC Current Limit) ---
    P_req_L = max(0, T_L * w_RL);
    P_req_R = max(0, T_R * w_RR);
    P_tot_req = P_req_L + P_req_R;
    
    P_limit_dc = V_dc * I_discharge_max;
    
    if P_tot_req > P_limit_dc
        scale_factor = P_limit_dc / P_tot_req;
        T_L = T_L * scale_factor;
        T_R = T_R * scale_factor;
    end
    
    % --- SATURAZIONE FINALE ---
    T_RL_cmd = max(-T_grip_max_RL, min(T_max_L, T_L));
    T_RR_cmd = max(-T_grip_max_RR, min(T_max_R, T_R));
end

== matlab function peacockElettricaSimulink/DriveController/Yaw_th/Bicycle Model Dynamic ==
  data: V input; yaw_th output; tan_delta input; wheelbase parameter; Kus parameter
function yaw_th = fcn(V,tan_delta,wheelbase,Kus)
% L = 1.55; %passo veicolo [m]
% yaw_th = (V / L) * tand;
%
  
yaw_th = (V / wheelbase) * tan_delta / (1 + Kus * V^2);



end

== matlab function peacockElettricaSimulink/DriveController/Yaw_th/tand safe ==
  data: tand input; tand_safe output; angle_limit_d parameter
function tand_safe = fcn(tand,angle_limit_d)
    soglia = tan(angle_limit_d*pi/180);  % 2° rad
    
    if abs(tand) < soglia
        tand_safe = 0;  % 
    else
        tand_safe = tand;  
    end
end

== matlab function peacockElettricaSimulink/DriveController/Yaw_th/yaw_saturation ==
  data: yaw_th input; yaw_sat output; V input; mu parameter; g parameter
function yaw_sat = fcn(yaw_th, V,mu, g)
    V_calc = max(V, 0.5);
    
    yaw_max_abs = (mu * g) / V_calc;
    yaw_sat = sign(yaw_th) * min(abs(yaw_th), yaw_max_abs);
end

== matlab function peacockElettricaSimulink/DriveController_/TVC/MATLAB Function1 ==
  data: dT_act input; dMz_act output; track_width parameter; R_wheel parameter; rid_ratio parameter; rid_eff parameter
function dMz_act = fcn(dT_act, track_width, R_wheel, rid_ratio, rid_eff)
    %Yaw moment (z) that the engines are currently delivering
    dMz_act = dT_act * track_width * rid_ratio * rid_eff / (2 * R_wheel);
end

== matlab function peacockElettricaSimulink/PeacockElettrica_/V ==
  data: Vx input; V output; Vy input
function V = fcn(Vx,Vy)

V = (Vx^2 + Vy^2)^0.5;

== stateflow chart peacockElettricaSimulink/DriveController_/Mode Manager ==
  state IDLE_
    entry:
    TVC_Target_Weight = 0;
  note: %[brake > 0 || (Throttle < tvc_throttle_on && V <= tvc_V_off)]
  state TVC_
    entry: TVC_Target_Weight = 1;
  (default) -> IDLE_
  TVC_ -> IDLE_ : [V <= tvc_V_off]
  IDLE_ -> TVC_ : [V > tvc_V_on]
  data: TVC_Target_Weight output; V input; D input; Throttle input; YawError input; brake input; tvc_D_thresh parameter; tvc_yaw_thresh parameter; tvc_yaw_thresh_off parameter; tvc_throttle_on parameter; tvc_V_on parameter; tvc_V_off parameter; tvc_D_thresh_off parameter

== matlab function peacockElettricaSimulink/G_motor_RL/Derating ==
  data: T_thermal input; T_req input; derating_out output; derating_prev input; derating_on_thresh parameter
function derating_out = fcn(T_thermal, T_req, derating_prev,derating_on_thresh)

if derating_prev == 0
    % Se NON sono in derating, controllo se devo entrarci
    if T_thermal < derating_on_thresh
        derating_out = 1;
    else
        derating_out = 0;
    end
else
    if T_req <= 1 % Uso un piccolo margine invece di 0 spaccato per robustezza numerica
        derating_out = 0; % Esco dal derating
    else
        derating_out = 1; % Mantengo il derating
    end
end
end
